simulink model "ECEN_5038_system_identiication_21Jan2020"  (R2019b)
settings: Solver=FixedStepAuto  StartTime=0.0  StopTime=10  FixedStep=.01  RelTol=1e-3
values from neighbouring files (symbols this model uses):
  a = 8    [ECEN_5038_21Jan2020.m]    (also in NAME_initialization_data.mat = 0.2; Quarc_Initialization.m = 0.2)
  k = 1    [ECEN_5038_21Jan2020.m]
  omega = 1    [ECEN_5038_21Jan2020.m]
  omega_range = freq_min:freq_min:freq_nyqist    [ECEN_5038_21Jan2020.m]
settings Model: Creator=Jack  LastModifiedBy=Jack

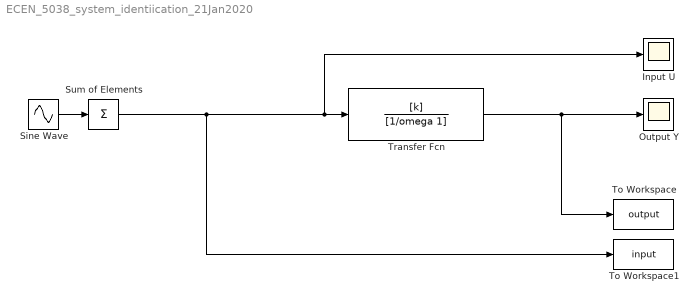
== system ECEN_5038_system_identiication_21Jan2020 ==
  Input U : Scope
      settings: Tag=Input U
  Output Y : Scope
  Sine Wave : Sin  Amplitude=a  Frequency=omega_range  SampleTime=0
  Sum of Elements : Sum  Inputs=+
  To Workspace : ToWorkspace  VariableName=output  SampleTime=-1
  To Workspace1 : ToWorkspace  VariableName=input  SampleTime=-1
  Transfer Fcn : TransferFcn  Numerator=[k]  Denominator=[1/omega 1]
  wires:
  Sine Wave/1 -> Sum of Elements/1
  Transfer Fcn/1 -> To Workspace/1, Output Y/1
  Sum of Elements/1 -> To Workspace1/1, Input U/1, Transfer Fcn/1
